simulink model "BehPackager"  (R2026a)
settings: Solver=VariableStepAuto
model workspace (MAT data in the model file):
  PackRate_bph = 200
  PackTau_s = 60
settings Model: DataDictionary=BehParamsCommon.sldd  ParameterArgumentNames=PackRate_bph,PackTau_s  Creator=sarah  LastModifiedBy=sarah

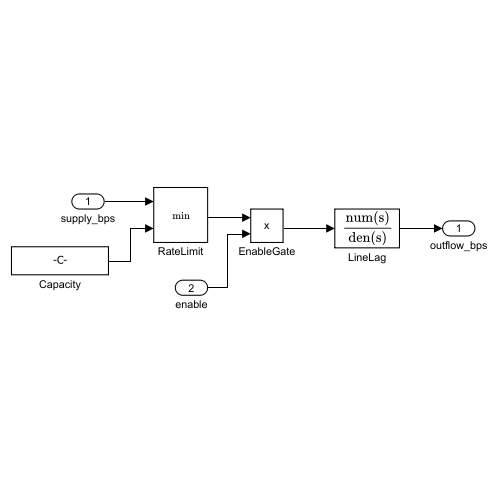
[thumbnail: Simulink's stored preview of the top-level diagram]
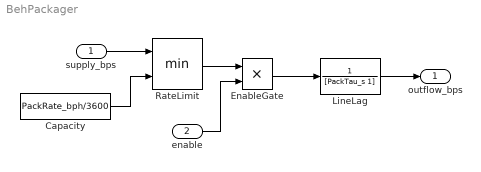
== system BehPackager ==
  supply_bps : Inport
  enable : Inport  Port=2
  Capacity : Constant  Value=PackRate_bph/3600
  EnableGate : Product
  LineLag : TransferFcn  Denominator=[PackTau_s 1]
  RateLimit : MinMax  Inputs=2
  outflow_bps : Outport
  wires:
  supply_bps/1 -> RateLimit/1
  Capacity/1 -> RateLimit/2
  RateLimit/1 -> EnableGate/1
  enable/1 -> EnableGate/2
  EnableGate/1 -> LineLag/1
  LineLag/1 -> outflow_bps/1
